simulink library "OpenManipulatorLib"  (R2017b)
settings: Solver=VariableStepAuto  StartTime=0.0  StopTime=10.0  RelTol=1e-3
undefined symbols (not defined in the file): ball_radius, eePositions, estDelay, filter_constant, gripper_force, initPosX, initPosY, initPosZ, initVelX, initVelY, initVelZ, polyOrder, time_jump, trajectoryPoints, Ts, wayPoints, X, Y, Z
libraries: sm_lib x85, nesl_utility x18, OpenManipulatorLib x11, fl_lib x4, Contact_Forces_Lib x3, dsppolyfun x2, Multibody_Multiphysics_Lib x2
(part 1 of 3)
settings Model: Creator=josea  LastModifiedBy=scastro

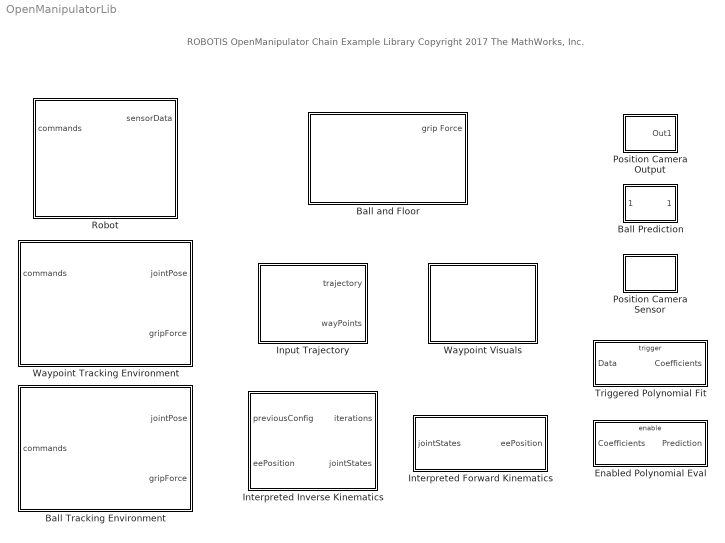
== system OpenManipulatorLib ==
  note: ROBOTIS OpenManipulator Chain Example Library
      |
      | Copyright 2017 The MathWorks, Inc.
  Ball Prediction : Subsystem  mask(Trajectory prediction in 2D){estDelay=estDelay, time_jump=time_jump, polyOrder=2}
      mask prompts: estDelay "Acquisition Window (seconds)"; time_jump "Time to look ahead (seconds)"; polyOrder "Polynomial Order"
      mask help: This subsystem estimates a polynomial using the data acquired until a specified time (estDelay), and then evaluates a polynomial with the calculated coefficients to give a rough prediction of where an object could be at a future point in time (time_jump).
      mask Display: image('PredictionIcon.png')
  Ball Tracking Environment : Subsystem  mask(Ball Tracking Environment){BallPositionY=-0.116, BallHeading=34.200, reverse=off, zVel=off}
      mask prompts: BallPositionY "Initial Ball Position (m)"; BallHeading "Initial Ball Heading (deg)"; reverse "Start from base and reverse heading"; zVel "3D Mode (Add Z initial velocity)"
      mask help: The initial position and velocity of the ball can be set to different conditions.
      mask init:
      | % Change the initial X position if the ball starting position is reversed
      | if ~reverse
      |     initPosX = 0.3;
      | else
      |     initPosX = 0;
      | end
      | 
      | % Initialize the ball velocity in XYZ coordinates
      | initPosY = BallPositionY;
      | VelocityMagnitude = 0.4;
      | initVelX = -1*VelocityMagnitude*cosd(BallHeading)*(-1)^reverse;
      | initVelY = VelocityMagnitude*sind(BallHeading);
      | initPosZ = 0.025;
      | if zVel
      |     initVelZ = 3.5;
      | else
      |     initVelZ = 0;
      | end
      mask Display: image('EnvironmentIcon.PNG')
  Ball and Floor : Subsystem  mask(Ball and Floor){PxPositionTargetValue=initPosX, PyPositionTargetValue=initPosY, PxVelocityTargetValue=initVelX, PyVelocityTargetValue=initVelY, PzPositionTargetValue=initPosZ, PzVelocityTargetValue=initVelZ}
      mask prompts: PxPositionTargetValue "Ball X Position Target"; PyPositionTargetValue "Ball Y Position Target"; PxVelocityTargetValue "Ball X Velocity Target"; PyVelocityTargetValue "Ball Y Velocity Target"; PzPositionTargetValue "Ball Z Position Target"; PzVelocityTargetValue "Ball Z Velocity Target"
      mask help: Subsystem containing ball and floor objects and the corresponding contact interfaces to interface with the manipulator gripper
      mask init:
      | if(any(PxVelocityTargetValue>0 || ...
      |        PyVelocityTargetValue>0 || ...
      |        PzVelocityTargetValue>0))
      |     stripColor = [1.0 0 1.0];
      | else
      |     stripColor = [0 0.6 0.6];
      | end
      mask TypeOptions PxPositionTargetValue: 6-DOF Joint/PxPositionTargetValue
      mask TypeOptions PyPositionTargetValue: 6-DOF Joint/PyPositionTargetValue
      mask TypeOptions PxVelocityTargetValue: 6-DOF Joint/PxVelocityTargetValue
      mask TypeOptions PyVelocityTargetValue: 6-DOF Joint/PyVelocityTargetValue
      mask TypeOptions PzPositionTargetValue: 6-DOF Joint/PzPositionTargetValue
      mask TypeOptions PzVelocityTargetValue: 6-DOF Joint/PzVelocityTargetValue
      mask Display: image('BallFloorIcon.png')
  Enabled Polynomial Eval : Subsystem
  Input Trajectory : Subsystem  mask(Input Trajectory){trajectorySelection=Simple}
      mask prompts: trajectorySelection "Trajectory type"
      mask help: This subsystem initializes data for the desired trajectory and waypoints. The necessary variables are created in the MATLAB workspace.
      mask init:
      | TS = get_param(gcb,'trajectorySelection');
      | switch TS
      |     case 'Simple'
      |         evalin('base','trajectorySelection=1;');
      |     case 'Complex'
      |         evalin('base','trajectorySelection=2;');
      |     case 'Gripper Fault'
      |         evalin('base','trajectorySelection=3;');
      | end
      | evalin('base','initOpenManipulatorWaypointTracking');
      mask TypeOptions trajectorySelection: Simple | Complex | Gripper Fault
      mask Display: image('wayPointsIcon.png')
  Interpreted Forward Kinematics : MATLAB Function  TreatAsAtomicUnit=on
  Interpreted Inverse Kinematics : MATLAB Function  TreatAsAtomicUnit=on
  Position Camera Output : Subsystem
      mask Display: image('CameraIcon.png')
  Position Camera Sensor : Subsystem
      mask Display: image('CameraIcon.png')
  Robot : Subsystem
      mask Display: image('RobotIcon.png')
  Triggered Polynomial Fit : Subsystem
  Waypoint Tracking Environment : Subsystem
      mask Display: image('EnvironmentWaypointsIcon.PNG')
  Waypoint Visuals : Subsystem  mask(Waypoint and Trajectory Visualization){spherePoints=wayPoints, sphereRadius=0.01, sphereColor=[0 0.5 1], splinePoints=trajectoryPoints, splineColor=[1 0 1]}
      mask prompts: spherePoints "Sphere Positions"; sphereRadius "Sphere Radius"; sphereColor "Sphere Color"; splinePoints "Trajectory Points"; splineColor "Trajectory Color"
      mask help:
      | This dynamic subsystem places spheres on the desired waypoints and visualizes a pre-computed trajectory as a 3D spline
      |
      | Sphere Positions and Trajectory Points are both vectors for which the first 3 columns correspond to the (X, Y, Z) coordinates of the waypoints or trajectory points.
      |
      | NOTE: Make sure the library link for the subsystem is broken when copied from the library. Otherwise the mask initialization will not be able to modify the subsystem contents.
      mask init:
      | % This initialization routine deletes everything within the mask except the
      | % inport and then rebuilds the subsystem with updated information from the
      | % mask parameters
      | 
      | subsystem = gcb;
      | blocks = find_system(subsystem,'LookUnderMasks','all');
      | 
      | % Delete all previous blocks except the inport
      | for idx = 2:length(blocks)-1
      |     delete_block(blocks{idx})
      | end
      | 
      | % Delete all signals
      | while ~isempty(find_system(subsystem,'LookUnderMasks','all','FindAll','on','type','line'))
      |     lines = find_system(subsystem,'LookUnderMasks','all','FindAll','on','type','line');
      |     delete_line(lines(1))
      | end
      | 
      | %%
      | pos1 = [140 100 180 140];
      | pos2 = [140 170 180 210];
      | 
      | set_param(strcat(subsystem,'/W'),'position',[140 60 180 80])
      | 
      | % Add spline to visualize trajectory
      | add_block('sm_lib/Curves and Surfaces/Spline',strcat(subsystem,'/Trajectory Spline'));
      | set_param(strcat(subsystem,'/Trajectory Spline'),'position',pos1,'Orientation','left');
      | set_param(strcat(subsystem,'/Trajectory Spline'),'DataPoints','splinePoints','EndCOnditionType','Natural','GraphicDiffuseColor','splineColor');
      | add_line(subsystem,strcat('W','/RConn1'),strcat('Trajectory Spline','/Lconn1'));
      | 
      | % Add waypoint sphere visuals
      | for idx = 1:size(spherePoints,1)
      |     pos1 = pos1 + [60 0 60 0];
      |     pos2 = pos2 + [60 0 60 0];
      |     
      |     % Add coordinate tranform and set parameters
      |     add_block('sm_lib/Frames and Transforms/Rigid Transform',strcat(subsystem,'/Rigid Transform',num2str(idx)));
      |     set_param(strcat(subsystem,'/Rigid Transform',num2str(idx)),'position',pos1,'Orientation','down');
      |     set_param(strcat(subsystem,'/Rigid Transform',num2str(idx)),'TranslationMethod','Cartesian','TranslationCartesianOffset',strcat('[',num2str(spherePoints(idx,1:3)),']'));
      |     add_line(subsystem,strcat('W','/RConn1'),strcat('Rigid Transform',num2str(idx),'/Lconn1'));
      |     
      |     % Add sphere ans set parameters
      |     add_block('sm_lib/Body Elements/Solid',strcat(subsystem,'/Solid',num2str(idx)))
      |     set_param(strcat(subsystem,'/Solid',num2str(idx)),'position',pos2,'GeometryShape','Sphere','GraphicDiffuseColor','sphereColor','SphereRadius','sphereRadius')
      |     add_line(subsystem,strcat('Rigid Transform',num2str(idx),'/Rconn1'),strcat('Solid',num2str(idx),'/RConn1'));
      |    
      | end
      mask DialogControl ParameterGroupVar Prompt: Sphere Parameters
      mask DialogControl Container3 Prompt: Spline Parameters
      mask Display: image('wayPointsIcon.png')

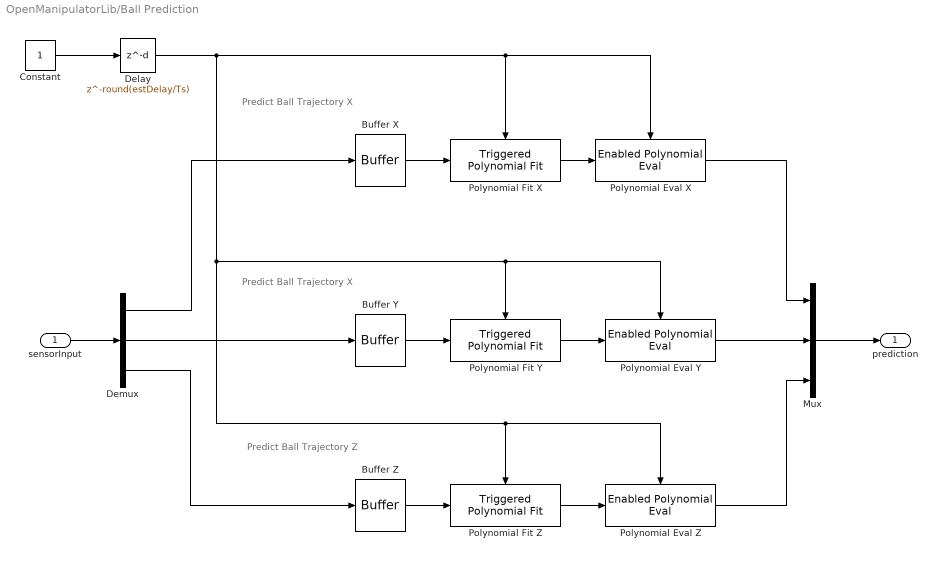
== system OpenManipulatorLib/Ball Prediction ==
  note: Predict Ball Trajectory X
  note: Predict Ball Trajectory X
  note: Predict Ball Trajectory Z
  sensorInput : Inport
  Buffer X : Buffer  N=round(estDelay/Ts)  V=round(estDelay/Ts)-1  OutputFrames=off
  Buffer Y : Buffer  N=round(estDelay/Ts)  V=round(estDelay/Ts)-1  OutputFrames=off
  Buffer Z : Buffer  N=round(estDelay/Ts)  V=round(estDelay/Ts)-1  OutputFrames=off
  Constant : Constant
  Delay : Delay  DelayLength=round(estDelay/Ts)
  Demux : Demux  Outputs=3
  Mux : Mux  Inputs=3
  Polynomial Eval X : OpenManipulatorLib/Enabled Polynomial Eval
  Polynomial Eval Y : OpenManipulatorLib/Enabled Polynomial Eval
  Polynomial Eval Z : OpenManipulatorLib/Enabled Polynomial Eval
  Polynomial Fit X : OpenManipulatorLib/Triggered Polynomial Fit
  Polynomial Fit Y : OpenManipulatorLib/Triggered Polynomial Fit
  Polynomial Fit Z : OpenManipulatorLib/Triggered Polynomial Fit
  prediction : Outport
  wires:
  Mux/1 -> prediction/1
  Constant/1 -> Delay/1
  sensorInput/1 -> Demux/1
  Demux/1 -> Buffer X/1
  Demux/2 -> Buffer Y/1
  Polynomial Eval X/1 -> Mux/1
  Delay/1 -> Polynomial Eval X/Enable, Polynomial Fit X/Trigger, Polynomial Eval Y/Enable, Polynomial Fit Y/Trigger, Polynomial Eval Z/Enable, Polynomial Fit Z/Trigger
  Polynomial Eval Z/1 -> Mux/3
  Demux/3 -> Buffer Z/1
  Buffer Z/1 -> Polynomial Fit Z/1
  Polynomial Fit Z/1 -> Polynomial Eval Z/1
  Polynomial Fit Y/1 -> Polynomial Eval Y/1
  Buffer Y/1 -> Polynomial Fit Y/1
  Buffer X/1 -> Polynomial Fit X/1
  Polynomial Fit X/1 -> Polynomial Eval X/1
  Polynomial Eval Y/1 -> Mux/2

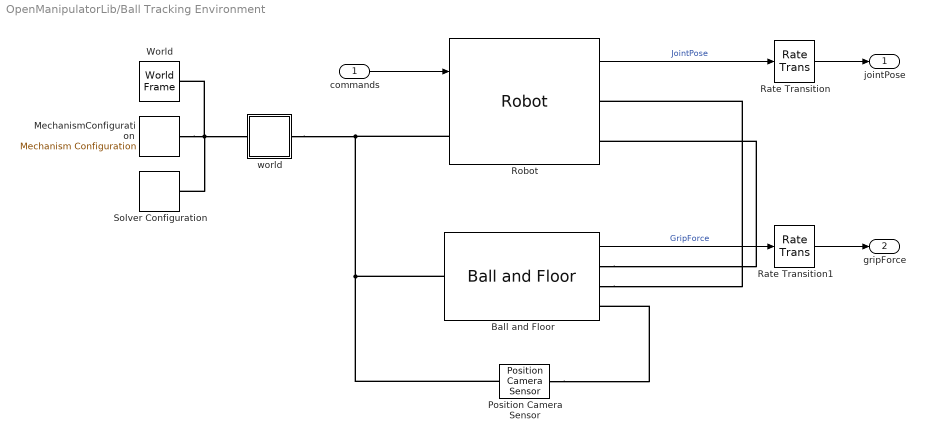
== system OpenManipulatorLib/Ball Tracking Environment ==
  commands : Inport
  Ball and Floor : OpenManipulatorLib/Ball and Floor  PxPositionTargetValue=initPosX  PyPositionTargetValue=initPosY  PxVelocityTargetValue=initVelX  PyVelocityTargetValue=initVelY  PzPositionTargetValue=initPosZ  PzVelocityTargetValue=initVelZ
  MechanismConfiguration : sm_lib/Utilities/Mechanism Configuration  UniformGravity=Constant  GravityVector=[0 0 -9.80665]  GravityUnits=m/s^2  LinearizationDelta=0.001
  Position Camera Sensor : OpenManipulatorLib/Position Camera Sensor  SystemSampleTime=-1
  Rate Transition : RateTransition
  Rate Transition1 : RateTransition
  Robot : OpenManipulatorLib/Robot  SystemSampleTime=-1
  Solver Configuration : nesl_utility/Solver Configuration  PhysicalDomain=network_engine_domain  SubClassName=solver  LeftPortType=input  RightPortType=generic  Accelerate=off  Tones=[]  Harmonics=[]  SimulateNoise=off  Profile=off  UseLocalSampling=off  EnableSwitchedLinearOptims=on  FrequencyDomain=off  UseCCode=off  RelTol=0.001  AbsTol=1e-06  MinStep=1e-09  ToWorkspace=off  RevertToSquareIcSolve=off  NumHomotopyIterations=100  PhasorMode=off  PhasorModeNumHarmonics=1  DoDC=off  ResidualTolerance=1e-09  UseLocalSolver=off  LocalSolverChoice=NE_BACKWARD_EULER_ADVANCER  LocalSolverSampleTime=0.001  DoFixedCost=off  MaxNonlinIter=3  MaxModeIter=2  LinearAlgebra=Sparse  DelaysMemoryBudget=1024  AutomaticFiltering=on  FilteringTimeConstant=0.001
  World : sm_lib/Frames and Transforms/World Frame
  world : Subsystem
  jointPose : Outport
  gripForce : Outport  Port=2
  wires:
  commands/1 -> Robot/1
  Robot/1 -> Rate Transition/1  "JointPose"
  Ball and Floor/1 -> Rate Transition1/1  "GripForce"
  Rate Transition/1 -> jointPose/1
  Rate Transition1/1 -> gripForce/1
  connections:
  World/RConn1 -- Solver Configuration/RConn1 -- world/LConn1 -- MechanismConfiguration/RConn1
  Position Camera Sensor/LConn1 -- Ball and Floor/LConn1 -- Robot/LConn1 -- world/RConn1
  Ball and Floor/RConn1 -- Robot/RConn2
  Ball and Floor/RConn2 -- Robot/RConn1
  Position Camera Sensor/RConn1 -- Ball and Floor/RConn3

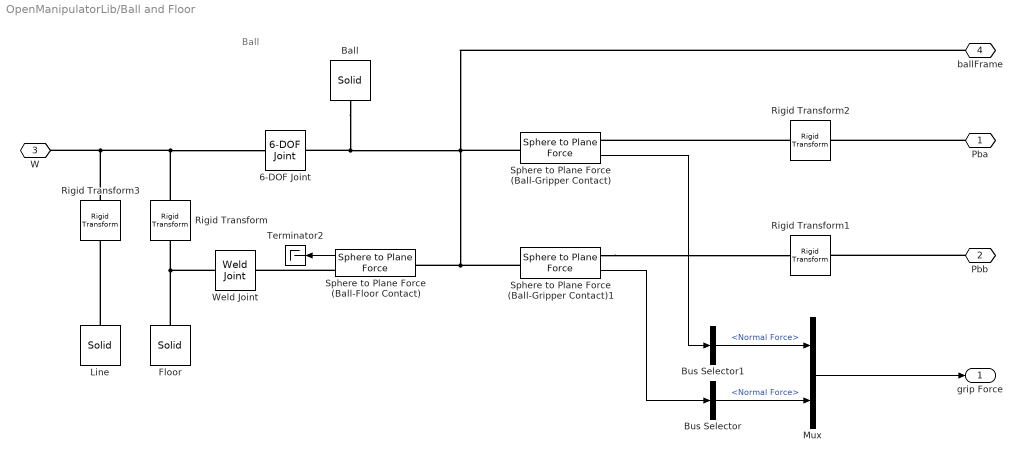
== system OpenManipulatorLib/Ball and Floor ==
  note: Ball
  6-DOF Joint : sm_lib/Joints/6-DOF Joint  SenseConstraintForce=off  SenseConstraintForceX=off  SenseConstraintForceY=off  SenseConstraintForceZ=off  SenseConstraintTorque=off  SenseConstraintTorqueX=off  SenseConstraintTorqueY=off  SenseConstraintTorqueZ=off  SenseTotalForce=off  SenseTotalForceX=off  SenseTotalForceY=off  SenseTotalForceZ=off  SenseTotalTorque=off  SenseTotalTorqueX=off  SenseTotalTorqueY=off  SenseTotalTorqueZ=off  CompositeWrenchDir=FollowerOnBase  CompositeWrenchFrame=BaseFrame  PxEquilibriumPosition=0  PxEquilibriumPositionUnits=m  PxSpringStiffness=0  PxSpringStiffnessUnits=N/m  PxDampingCoefficient=contact_floor.dampingCoeff  PxDampingCoefficientUnits=N/(m/s)  PxTorqueActuationMode=NoTorque  PxMotionActuationMode=ComputedMotion  PxSensePosition=off  PxSenseVelocity=off  PxSenseAcceleration=off  PxSenseTorqueForce=off  PxPositionTargetSpecify=on  PxPositionTargetPriority=High  PxPositionTargetValue=PxPositionTargetValue  PxPositionTargetValueUnits=m  PxVelocityTargetSpecify=on  PxVelocityTargetPriority=High  PxVelocityTargetValue=PxVelocityTargetValue  PxVelocityTargetValueUnits=m/s  PyEquilibriumPosition=0  PyEquilibriumPositionUnits=m  PySpringStiffness=0  PySpringStiffnessUnits=N/m  PyDampingCoefficient=contact_floor.dampingCoeff  PyDampingCoefficientUnits=N/(m/s)  PyTorqueActuationMode=NoTorque  PyMotionActuationMode=ComputedMotion  PySensePosition=off  PySenseVelocity=off  PySenseAcceleration=off  PySenseTorqueForce=off  PyPositionTargetSpecify=on  PyPositionTargetPriority=High  PyPositionTargetValue=PyPositionTargetValue  PyPositionTargetValueUnits=m  PyVelocityTargetSpecify=on  PyVelocityTargetPriority=High  PyVelocityTargetValue=PyVelocityTargetValue  PyVelocityTargetValueUnits=m/s  PzEquilibriumPosition=0  PzEquilibriumPositionUnits=m  PzSpringStiffness=0  PzSpringStiffnessUnits=N/m  PzDampingCoefficient=0  PzDampingCoefficientUnits=N/(m/s)  PzTorqueActuationMode=NoTorque  PzMotionActuationMode=ComputedMotion  PzSensePosition=off  PzSenseVelocity=off  PzSenseAcceleration=off  PzSenseTorqueForce=off  PzPositionTargetSpecify=on  PzPositionTargetPriority=High  PzPositionTargetValue=PzPositionTargetValue  PzPositionTargetValueUnits=m  PzVelocityTargetSpecify=on  PzVelocityTargetPriority=High  PzVelocityTargetValue=PzVelocityTargetValue  PzVelocityTargetValueUnits=m/s  SphDefPosRotationMethod=None  SphDefPosRotationAngleUnits=deg  SphDefPosRotationStandardAxis=+Z  SphDefPosRotationAngle=0.0  SphDefPosRotationArbitraryAxis=[0 0 1]  SphDefPosFollAlignAxisA=+X  SphDefPosBaseAlignAxisA=+Y  SphDefPosFollAlignAxisB=+Y  SphDefPosBaseAlignAxisB=+Z  SphDefPosRotationSequenceAxes=FollowerAxes  SphDefPosRotationSequence=XYX  SphDefPosRotationSequenceAngles=[0 0 0]  SphDefPosRotationSequenceAnglesUnits=deg  SphDefPosRotationMatrix=[1 0 0; 0 1 0; 0 0 1]  SphEqPosRotationMethod=None  SphEqPosRotationAngleUnits=deg  SphEqPosRotationStandardAxis=+Z  SphEqPosRotationAngle=0.0  SphEqPosRotationArbitraryAxis=[0 0 1]  SphEqPosFollAlignAxisA=+X  SphEqPosBaseAlignAxisA=+Y  SphEqPosFollAlignAxisB=+Y  SphEqPosBaseAlignAxisB=+Z  SphEqPosRotationSequenceAxes=FollowerAxes  SphEqPosRotationSequence=XYX  SphEqPosRotationSequenceAngles=[0 0 0]  SphEqPosRotationSequenceAnglesUnits=deg  SphEqPosRotationMatrix=[1 0 0; 0 1 0; 0 0 1]  SphSpringStiffness=0  SphSpringStiffnessUnits=N*m/deg  SphDampingCoefficient=contact_floor.dampingCoeffR  SphDampingCoefficientUnits=N*m/(rad/s)  SphActuateTorqueX=off  SphActuateTorqueY=off  SphActuateTorqueZ=off  SphActuateTorque=off  SphTorqueActuationMode=NoTorque  SphMotionActuationMode=ComputedMotion  SphActuationFrame=BaseFrame  SphSensePosition=off  SphSenseVelocityX=off  SphSenseVelocityY=off  SphSenseVelocityZ=off  SphSenseVelocity=off  SphSenseAccelerationX=off  SphSenseAccelerationY=off  SphSenseAccelerationZ=off  SphSenseAcceleration=off  SphSenseTorqueX=off  SphSenseTorqueY=off  SphSenseTorqueZ=off  SphSenseTorqueForce=off  SphSensingFrame=BaseFrame  SphPositionTargetRotationMethod=None  SphPositionTargetRotationAngleUnits=deg  SphPositionTargetRotationStandardAxis=+Z  SphPositionTargetRotationAngle=0.0  SphPositionTargetRotationArbitraryAxis=[0 0 1]  SphPositionTargetFollAlignAxisA=+X  SphPositionTargetBaseAlignAxisA=+Y  SphPositionTargetFollAlignAxisB=+Y  SphPositionTargetBaseAlignAxisB=+Z  SphPositionTargetRotationSequenceAxes=FollowerAxes  SphPositionTargetRotationSequence=XYX  SphPositionTargetRotationSequenceAngles=[0 0 0]  SphPositionTargetRotationSequenceAnglesUnits=deg  SphPositionTargetRotationMatrix=[1 0 0; 0 1 0; 0 0 1]  SphPositionTargetSpecify=off  SphPositionTargetPriority=High  SphVelocityTargetValue=[0 0 0]  SphVelocityTargetValueUnits=deg/s  SphVelocityTargetSpecify=off  SphVelocityTargetPriority=High  SphVelocityTargetInFollowerFrame=on
  Ball : sm_lib/Body Elements/Solid  InertiaType=CalculateFromGeometry  Mass=0.01  MassUnits=kg  CenterOfMass=[0 0 0]  CenterOfMassUnits=m  MomentsOfInertia=[1 1 1]  MomentsOfInertiaUnits=kg*m^2  ProductsOfInertia=[1 1 1]  ProductsOfInertiaUnits=kg*m^2  DensityBased=off  Density=1000  DensityUnits=kg/m^3  DoExposeReferenceFrame=on  SerializedFrames=<Frames/>  GraphicType=FromGeometry  MarkerShape=Sphere  MarkerSize=10  GraphicVisPropType=SimpleVisualProperties  GraphicDiffuseColor=[1.0 0.2 0.2]  GraphicSpecularColor=[0.5 0.5 0.5 1.0]  GraphicAmbientColor=[0.15 0.15 0.15 1.0]  GraphicEmissiveColor=[0.0 0.0 0.0 1.0]  GraphicShininess=75  GraphicOpacity=1.0  GeometryShape=Sphere  RectangleSize=[1 1]  RectangleSizeUnits=m  BrickDimensions=[40 40 0.5]  BrickDimensionUnits=cm  CylinderRadius=1  CylinderRadiusUnits=m  CylinderLength=1  CylinderLengthUnits=m  SphereRadius=ball_radius  SphereRadiusUnits=cm  EllipsoidRadii=[1 1 1]  EllipsoidRadiiUnits=m  ExtrusionCrossSection=[1 1; -1 1; -1 -1; 1 -1]  ExtrusionCrossSectionUnits=m  ExtrusionLength=1  ExtrusionLengthUnits=m  PolygonNumSides=3  PolygonOuterRadius=1  PolygonOuterRadiusUnits=m  ExtGeomFileType=STEP  ExtGeomFileUnits=m  RevolutionCrossSection=[1 1; 1 -1; 2 -1; 2 1]  RevolutionCrossSectionUnits=m  RevolutionExtent=Full  RevolutionAngle=180  RevolutionAngleUnits=deg
  Bus Selector : BusSelector  OutputSignals=Normal Force
  Bus Selector1 : BusSelector  OutputSignals=Normal Force
  Floor : sm_lib/Body Elements/Solid  InertiaType=CalculateFromGeometry  Mass=1  MassUnits=kg  CenterOfMass=[0 0 0]  CenterOfMassUnits=m  MomentsOfInertia=[1 1 1]  MomentsOfInertiaUnits=kg*m^2  ProductsOfInertia=[1 1 1]  ProductsOfInertiaUnits=kg*m^2  DensityBased=on  Density=1000  DensityUnits=kg/m^3  DoExposeReferenceFrame=on  SerializedFrames=<Frames/>  GraphicType=FromGeometry  MarkerShape=Sphere  MarkerSize=10  GraphicVisPropType=SimpleVisualProperties  GraphicDiffuseColor=[0.0 0.6 0.6]  GraphicSpecularColor=[0.5 0.5 0.5 1.0]  GraphicAmbientColor=[0.15 0.15 0.15 1.0]  GraphicEmissiveColor=[0.0 0.0 0.0 1.0]  GraphicShininess=75  GraphicOpacity=1.0  GeometryShape=Brick  RectangleSize=[1 1]  RectangleSizeUnits=m  BrickDimensions=floor_dimensions  BrickDimensionUnits=cm  CylinderRadius=1  CylinderRadiusUnits=m  CylinderLength=1  CylinderLengthUnits=m  SphereRadius=1  SphereRadiusUnits=m  EllipsoidRadii=[1 1 1]  EllipsoidRadiiUnits=m  ExtrusionCrossSection=[1 1; -1 1; -1 -1; 1 -1]  ExtrusionCrossSectionUnits=m  ExtrusionLength=1  ExtrusionLengthUnits=m  PolygonNumSides=3  PolygonOuterRadius=1  PolygonOuterRadiusUnits=m  ExtGeomFileType=STEP  ExtGeomFileUnits=m  RevolutionCrossSection=[1 1; 1 -1; 2 -1; 2 1]  RevolutionCrossSectionUnits=m  RevolutionExtent=Full  RevolutionAngle=180  RevolutionAngleUnits=deg
  Line : sm_lib/Body Elements/Solid  InertiaType=CalculateFromGeometry  Mass=1  MassUnits=kg  CenterOfMass=[0 0 0]  CenterOfMassUnits=m  MomentsOfInertia=[1 1 1]  MomentsOfInertiaUnits=kg*m^2  ProductsOfInertia=[1 1 1]  ProductsOfInertiaUnits=kg*m^2  DensityBased=on  Density=1000  DensityUnits=kg/m^3  DoExposeReferenceFrame=on  SerializedFrames=<Frames/>  GraphicType=FromGeometry  MarkerShape=Sphere  MarkerSize=10  GraphicVisPropType=SimpleVisualProperties  GraphicDiffuseColor=stripColor  GraphicSpecularColor=[0.5 0.5 0.5 1.0]  GraphicAmbientColor=[0.15 0.15 0.15 1.0]  GraphicEmissiveColor=[0.0 0.0 0.0 1.0]  GraphicShininess=75  GraphicOpacity=1.0  GeometryShape=Brick  RectangleSize=[1 1]  RectangleSizeUnits=m  BrickDimensions=[1 40 0.505]  BrickDimensionUnits=cm  CylinderRadius=1  CylinderRadiusUnits=m  CylinderLength=1  CylinderLengthUnits=m  SphereRadius=1  SphereRadiusUnits=m  EllipsoidRadii=[1 1 1]  EllipsoidRadiiUnits=m  ExtrusionCrossSection=[1 1; -1 1; -1 -1; 1 -1]  ExtrusionCrossSectionUnits=m  ExtrusionLength=1  ExtrusionLengthUnits=m  PolygonNumSides=3  PolygonOuterRadius=1  PolygonOuterRadiusUnits=m  ExtGeomFileType=STEP  ExtGeomFileUnits=m  RevolutionCrossSection=[1 1; 1 -1; 2 -1; 2 1]  RevolutionCrossSectionUnits=m  RevolutionExtent=Full  RevolutionAngle=180  RevolutionAngleUnits=deg
  Mux : Mux  Inputs=2
  Rigid Transform : sm_lib/Frames and Transforms/Rigid Transform  TranslationMethod=Cartesian  TranslationStandardOffset=0  TranslationLengthUnit=cm  TranslationStandardAxis=+Z  TranslationCartesianOffset=[15 0 -0.25]  TranslationROffset=0  TranslationROffsetUnits=m  TranslationZOffset=0  TranslationZOffsetUnits=m  TranslationThetaOffset=0  TranslationThetaOffsetUnits=deg  RotationMethod=None  RotationAngleUnits=deg  RotationStandardAxis=+Z  RotationAngle=0.0  RotationArbitraryAxis=[0 0 1]  FollAlignAxisA=+X  BaseAlignAxisA=+Y  FollAlignAxisB=+Y  BaseAlignAxisB=+Z  RotationSequenceAxes=FollowerAxes  RotationSequence=XYX  RotationSequenceAngles=[0 0 0]  RotationSequenceAnglesUnits=deg  RotationMatrix=[1 0 0; 0 1 0; 0 0 1]
  Rigid Transform1 : sm_lib/Frames and Transforms/Rigid Transform  TranslationMethod=None  TranslationStandardOffset=0  TranslationLengthUnit=cm  TranslationStandardAxis=+Z  TranslationCartesianOffset=[15 0 -0.25]  TranslationROffset=0  TranslationROffsetUnits=m  TranslationZOffset=0  TranslationZOffsetUnits=m  TranslationThetaOffset=0  TranslationThetaOffsetUnits=deg  RotationMethod=StandardAxis  RotationAngleUnits=deg  RotationStandardAxis=+X  RotationAngle=-90  RotationArbitraryAxis=[0 0 1]  FollAlignAxisA=+X  BaseAlignAxisA=+Y  FollAlignAxisB=+Y  BaseAlignAxisB=+Z  RotationSequenceAxes=FollowerAxes  RotationSequence=XYX  RotationSequenceAngles=[0 0 0]  RotationSequenceAnglesUnits=deg  RotationMatrix=[1 0 0; 0 1 0; 0 0 1]
  Rigid Transform2 : sm_lib/Frames and Transforms/Rigid Transform  TranslationMethod=None  TranslationStandardOffset=0  TranslationLengthUnit=cm  TranslationStandardAxis=+Z  TranslationCartesianOffset=[15 0 -0.25]  TranslationROffset=0  TranslationROffsetUnits=m  TranslationZOffset=0  TranslationZOffsetUnits=m  TranslationThetaOffset=0  TranslationThetaOffsetUnits=deg  RotationMethod=StandardAxis  RotationAngleUnits=deg  RotationStandardAxis=+X  RotationAngle=-90  RotationArbitraryAxis=[0 0 1]  FollAlignAxisA=+X  BaseAlignAxisA=+Y  FollAlignAxisB=+Y  BaseAlignAxisB=+Z  RotationSequenceAxes=FollowerAxes  RotationSequence=XYX  RotationSequenceAngles=[0 0 0]  RotationSequenceAnglesUnits=deg  RotationMatrix=[1 0 0; 0 1 0; 0 0 1]
  Rigid Transform3 : sm_lib/Frames and Transforms/Rigid Transform  TranslationMethod=Cartesian  TranslationStandardOffset=0  TranslationLengthUnit=cm  TranslationStandardAxis=+Z  TranslationCartesianOffset=[30 0 -0.25]  TranslationROffset=0  TranslationROffsetUnits=m  TranslationZOffset=0  TranslationZOffsetUnits=m  TranslationThetaOffset=0  TranslationThetaOffsetUnits=deg  RotationMethod=None  RotationAngleUnits=deg  RotationStandardAxis=+Z  RotationAngle=0.0  RotationArbitraryAxis=[0 0 1]  FollAlignAxisA=+X  BaseAlignAxisA=+Y  FollAlignAxisB=+Y  BaseAlignAxisB=+Z  RotationSequenceAxes=FollowerAxes  RotationSequence=XYX  RotationSequenceAngles=[0 0 0]  RotationSequenceAnglesUnits=deg  RotationMatrix=[1 0 0; 0 1 0; 0 0 1]
  Sphere to Plane Force (Ball-Floor Contact) : Contact_Forces_Lib/3D/Sphere to Plane Force  sphere_rad=ball_radius*0.01  plane_lenx=contact_floor.planeLength  plane_leny=contact_floor.planeLength  plane_depth=contact_floor.planeDepth  force_law=Linear  k_contact=contact_floor.stiffness  b_contact=contact_floor.damping  pen_full_damp_F=1e-4  pen_exponent=2  custom_param_1=1  custom_param_2=1  friction_law=Stick-Slip Continuous  mu_kinetic=contact_floor.kFrictionCoeff  mu_static=contact_floor.sFrictionCoeff  v_thr=0.01  vis_on=off  vis_opc_en=0  vis_len_plaBz=0.005  vis_clr=[0.9 0.2 0.2]  vis_opc=0.7
  Sphere to Plane Force (Ball-Gripper Contact) : Contact_Forces_Lib/3D/Sphere to Plane Force  sphere_rad=ball_radius*0.01  plane_lenx=contact_gripper.planeLength_x  plane_leny=contact_gripper.planeLength_y  plane_depth=contact_gripper.planeDepth  force_law=Linear  k_contact=contact_gripper.stiffness  b_contact=contact_gripper.damping  pen_full_damp_F=1e-4  pen_exponent=1  custom_param_1=1  custom_param_2=1  friction_law=Stick-Slip Continuous  mu_kinetic=contact_gripper.kFrictionCoeff  mu_static=contact_gripper.sFrictionCoeff  v_thr=0.01  vis_on=off  vis_opc_en=0  vis_len_plaBz=0.005  vis_clr=[0.9 0.2 0.2]  vis_opc=0.7
  Sphere to Plane Force (Ball-Gripper Contact)1 : Contact_Forces_Lib/3D/Sphere to Plane Force  sphere_rad=ball_radius*0.01  plane_lenx=contact_gripper.planeLength_x  plane_leny=contact_gripper.planeLength_y  plane_depth=contact_gripper.planeDepth  force_law=Linear  k_contact=contact_gripper.stiffness  b_contact=contact_gripper.damping  pen_full_damp_F=1e-4  pen_exponent=1  custom_param_1=1  custom_param_2=1  friction_law=Stick-Slip Continuous  mu_kinetic=contact_gripper.kFrictionCoeff  mu_static=contact_gripper.sFrictionCoeff  v_thr=0.01  vis_on=off  vis_opc_en=0  vis_len_plaBz=0.005  vis_clr=[0.9 0.2 0.2]  vis_opc=0.7
  Terminator2 : Terminator
  Weld Joint : sm_lib/Joints/Weld Joint  SenseConstraintForce=off  SenseConstraintForceX=off  SenseConstraintForceY=off  SenseConstraintForceZ=off  SenseConstraintTorque=off  SenseConstraintTorqueX=off  SenseConstraintTorqueY=off  SenseConstraintTorqueZ=off  SenseTotalForce=off  SenseTotalForceX=off  SenseTotalForceY=off  SenseTotalForceZ=off  SenseTotalTorque=off  SenseTotalTorqueX=off  SenseTotalTorqueY=off  SenseTotalTorqueZ=off  CompositeWrenchDir=FollowerOnBase  CompositeWrenchFrame=BaseFrame
  Pba : PMIOPort  Port=1  Side=Right
  Pbb : PMIOPort  Port=2  Side=Right
  W : PMIOPort  Port=3  Side=Left
  ballFrame : PMIOPort  Port=4  Side=Right
  grip Force : Outport
  wires:
  Sphere to Plane Force (Ball-Gripper Contact)1/1 -> Bus Selector/1
  Sphere to Plane Force (Ball-Floor Contact)/1 -> Terminator2/1
  Sphere to Plane Force (Ball-Gripper Contact)/1 -> Bus Selector1/1
  Bus Selector1/1 -> Mux/1  "<Normal Force>"
  Bus Selector/1 -> Mux/2  "<Normal Force>"
  Mux/1 -> grip Force/1
  connections:
  Floor/RConn1 -- Weld Joint/LConn1 -- Rigid Transform/RConn1
  Pba/RConn1 -- Rigid Transform2/LConn1
  6-DOF Joint/RConn1 -- Sphere to Plane Force (Ball-Gripper Contact)/LConn1 -- ballFrame/RConn1 -- Sphere to Plane Force (Ball-Gripper Contact)1/LConn1 -- Sphere to Plane Force (Ball-Floor Contact)/LConn1 -- Ball/RConn1
  Pbb/RConn1 -- Rigid Transform1/LConn1
  Sphere to Plane Force (Ball-Gripper Contact)1/RConn1 -- Rigid Transform1/RConn1
  Sphere to Plane Force (Ball-Floor Contact)/RConn1 -- Weld Joint/RConn1
  Rigid Transform2/RConn1 -- Sphere to Plane Force (Ball-Gripper Contact)/RConn1
  Rigid Transform/LConn1 -- Rigid Transform3/LConn1 -- W/RConn1 -- 6-DOF Joint/LConn1
  Line/RConn1 -- Rigid Transform3/RConn1

== system OpenManipulatorLib/Enabled Polynomial Eval ==
  Coefficients : Inport
  Enable : EnablePort
  Add : Sum
  Clock : Clock
  Constant : Constant  Value=time_jump
  Polynomial Evaluation : dsppolyfun/Polynomial Evaluation  useConstCoeffs=off  constCoeffs=[5 4 3 2 1]
      settings: SourceProductName=DSP System Toolbox  SourceProductBaseCode=DS
  Rate Transition : RateTransition  OutPortSampleTime=Ts
  Prediction : Outport
  wires:
  Polynomial Evaluation/1 -> Prediction/1
  Add/1 -> Polynomial Evaluation/1
  Constant/1 -> Add/2
  Rate Transition/1 -> Add/1
  Coefficients/1 -> Polynomial Evaluation/2
  Clock/1 -> Rate Transition/1

== system OpenManipulatorLib/Input Trajectory ==
  Constant : Constant  Value=eePositions
  Constant3 : Constant  Value=wayPoints
  trajectory : Outport
  wayPoints : Outport  Port=2
  wires:
  Constant/1 -> trajectory/1
  Constant3/1 -> wayPoints/1

== system OpenManipulatorLib/Position Camera Output ==
  Mux : Mux  Inputs=3
  Out1 : Outport
  wires:
  [ballX] -> Mux/1
  [ballY] -> Mux/2
  Mux/1 -> Out1/1
  [ballZ] -> Mux/3

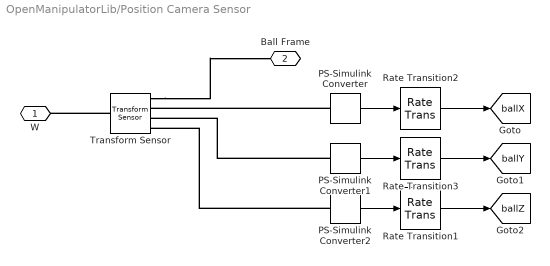
== system OpenManipulatorLib/Position Camera Sensor ==
  PS-Simulink Converter : nesl_utility/PS-Simulink Converter  PhysicalDomain=network_engine_domain  SubClassName=ps_output  LeftPortType=input  RightPortType=output  PseudoPeriodic=off  Frequencies=[]  Unit=1  AffineConversion=off
  PS-Simulink Converter1 : nesl_utility/PS-Simulink Converter  PhysicalDomain=network_engine_domain  SubClassName=ps_output  LeftPortType=input  RightPortType=output  PseudoPeriodic=off  Frequencies=[]  Unit=1  AffineConversion=off
  PS-Simulink Converter2 : nesl_utility/PS-Simulink Converter  PhysicalDomain=network_engine_domain  SubClassName=ps_output  LeftPortType=input  RightPortType=output  PseudoPeriodic=off  Frequencies=[]  Unit=1  AffineConversion=off
  Rate Transition1 : RateTransition  OutPortSampleTime=Ts
  Rate Transition2 : RateTransition  OutPortSampleTime=Ts
  Rate Transition3 : RateTransition  OutPortSampleTime=Ts
  Transform Sensor : sm_lib/Frames and Transforms/Transform Sensor  MeasurementFrame=World  SenseAngle=off  SenseAxis=off  SenseAngle1=off  SenseAngle2=off  SenseAngle3=off  SenseQ=off  SenseR=off  SenseOmegaX=off  SenseOmegaY=off  SenseOmegaZ=off  SenseOmega1=off  SenseOmega2=off  SenseOmega3=off  SenseQDot=off  SenseRDot=off  SenseAlphaX=off  SenseAlphaY=off  SenseAlphaZ=off  SenseAlpha1=off  SenseAlpha2=off  SenseAlpha3=off  SenseQDDot=off  SenseRDDot=off  SenseX=on  SenseY=on  SenseZ=on  SenseRad=off  SenseAzim=off  SenseDist=off  SenseInc=off  SenseXDot=off  SenseYDot=off  SenseZDot=off  SenseRadDot=off  SenseAzimDot=off  SenseDistDot=off  SenseIncDot=off  SenseXDDot=off  SenseYDDot=off  SenseZDDot=off  SenseRadDDot=off  SenseAzimDDot=off  SenseDistDDot=off  SenseIncDDot=off
  W : PMIOPort  Port=1  Side=Left
  Ball Frame : PMIOPort  Port=2  Side=Right
  tag scope: ballX=global, ballY=global, ballZ=global
  wires:
  PS-Simulink Converter1/1 -> Rate Transition3/1
  PS-Simulink Converter/1 -> Rate Transition2/1
  Rate Transition2/1 -> [ballX]
  Rate Transition3/1 -> [ballY]
  Rate Transition1/1 -> [ballZ]
  PS-Simulink Converter2/1 -> Rate Transition1/1
  connections:
  PS-Simulink Converter/LConn1 -- Transform Sensor/RConn2
  PS-Simulink Converter1/LConn1 -- Transform Sensor/RConn3
  Transform Sensor/LConn1 -- W/RConn1
  Transform Sensor/RConn1 -- Ball Frame/RConn1
  PS-Simulink Converter2/LConn1 -- Transform Sensor/RConn4

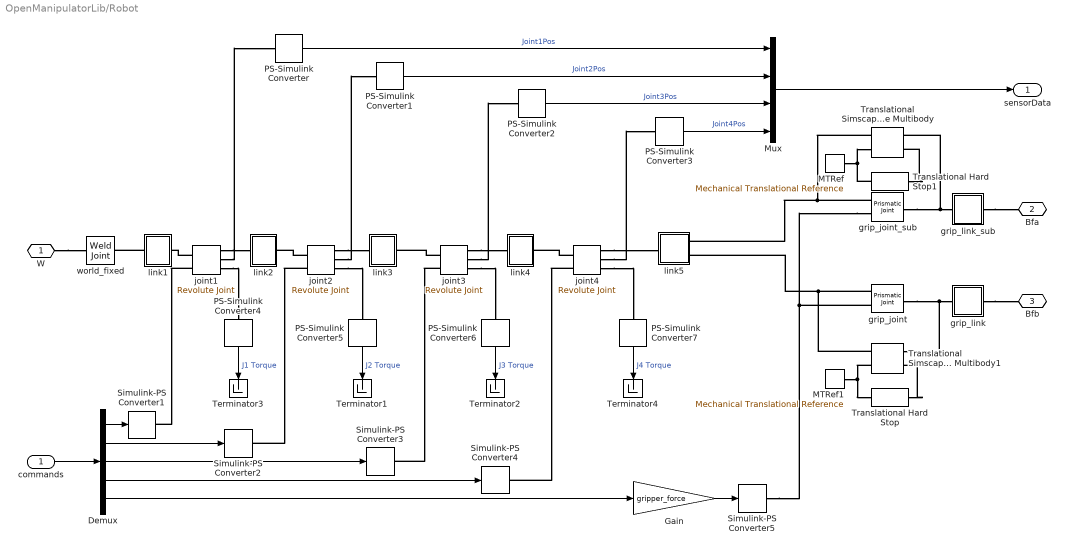
== system OpenManipulatorLib/Robot ==
  commands : Inport
  Demux : Demux  Outputs=5
  Gain : Gain  Gain=gripper_force
  MTRef : fl_lib/Mechanical/Translational Elements/Mechanical Translational Reference
  MTRef1 : fl_lib/Mechanical/Translational Elements/Mechanical Translational Reference
  Mux : Mux
  PS-Simulink Converter{,1..7} (8 alike) : nesl_utility/PS-Simulink Converter  PhysicalDomain=network_engine_domain  SubClassName=ps_output  LeftPortType=input  RightPortType=output  PseudoPeriodic=off  Frequencies=[]  Unit=1  AffineConversion=off
  Simulink-PS Converter{1..4} (4 alike) : nesl_utility/Simulink-PS Converter  PhysicalDomain=network_engine_domain  SubClassName=ps_input  LeftPortType=input  RightPortType=output  PseudoPeriodic=off  Frequencies=[]  NoiseDistribution=none  NoiseParameters=[]  Unit=1  AffineConversion=off  FilteringAndDerivatives=filter  SimscapeFilterOrder=2  InputFilterTimeConstant=filter_constant  UdotUserProvided=0
  Simulink-PS Converter5 : nesl_utility/Simulink-PS Converter  PhysicalDomain=network_engine_domain  SubClassName=ps_input  LeftPortType=input  RightPortType=output  PseudoPeriodic=off  Frequencies=[]  NoiseDistribution=none  NoiseParameters=[]  Unit=1  AffineConversion=off  FilteringAndDerivatives=filter  SimscapeFilterOrder=2  InputFilterTimeConstant=filter_constant*0.1  UdotUserProvided=0
  Terminator{1..4} (4 alike) : Terminator
  Translational Simscape Multibody : Multibody_Multiphysics_Lib/Interfaces/Translational Simscape Multibody
      settings: SourceProductName=Simscape Multibody Multiphysics Library
  Translational Simscape Multibody1 : Multibody_Multiphysics_Lib/Interfaces/Translational Simscape Multibody
      settings: SourceProductName=Simscape Multibody Multiphysics Library
  Translational Hard Stop : fl_lib/Mechanical/Translational Elements/Translational Hard Stop  upper_bnd=0.01 m  lower_bnd=-0.03 m  stiff_up=1e6 N/m  stiff_low=1e6 N/m  D_up=150 N/(m/s)  D_low=150 N/(m/s)  model=1  transition=0.1 mm  v_specify=off  v_priority=None  v=0 m/s  v_nominal_specify=off  v_nominal_unit=m/s  v_nominal_value=1  f_specify=off  f_priority=None  f=0 N  f_nominal_specify=off  f_nominal_unit=N  f_nominal_value=1  x_specify=off  x_priority=High  x=0 m  x_nominal_specify=off  x_nominal_unit=m  x_nominal_value=1
  Translational Hard Stop1 : fl_lib/Mechanical/Translational Elements/Translational Hard Stop  upper_bnd=0.01 m  lower_bnd=-0.03 m  stiff_up=1e6 N/m  stiff_low=1e6 N/m  D_up=150 N/(m/s)  D_low=150 N/(m/s)  model=1  transition=0.1 mm  v_specify=off  v_priority=None  v=0 m/s  v_nominal_specify=off  v_nominal_unit=m/s  v_nominal_value=1  f_specify=off  f_priority=None  f=0 N  f_nominal_specify=off  f_nominal_unit=N  f_nominal_value=1  x_specify=off  x_priority=High  x=0 m  x_nominal_specify=off  x_nominal_unit=m  x_nominal_value=1
  grip_joint : sm_lib/Joints/Prismatic Joint  SenseConstraintForce=off  SenseConstraintForceX=off  SenseConstraintForceY=off  SenseConstraintForceZ=off  SenseConstraintTorque=off  SenseConstraintTorqueX=off  SenseConstraintTorqueY=off  SenseConstraintTorqueZ=off  SenseTotalForce=off  SenseTotalForceX=off  SenseTotalForceY=off  SenseTotalForceZ=off  SenseTotalTorque=off  SenseTotalTorqueX=off  SenseTotalTorqueY=off  SenseTotalTorqueZ=off  CompositeWrenchDir=FollowerOnBase  CompositeWrenchFrame=BaseFrame  EquilibriumPosition=0  EquilibriumPositionUnits=m  SpringStiffness=1  SpringStiffnessUnits=N/m  DampingCoefficient=5  DampingCoefficientUnits=kg/s  TorqueActuationMode=InputTorque  MotionActuationMode=ComputedMotion  SensePosition=off  SenseVelocity=off  SenseAcceleration=off  SenseTorqueForce=off  PositionTargetSpecify=off  PositionTargetPriority=High  PositionTargetValue=0  PositionTargetValueUnits=m  VelocityTargetSpecify=off  VelocityTargetPriority=High  VelocityTargetValue=0  VelocityTargetValueUnits=m/s
  grip_joint_sub : sm_lib/Joints/Prismatic Joint  SenseConstraintForce=off  SenseConstraintForceX=off  SenseConstraintForceY=off  SenseConstraintForceZ=off  SenseConstraintTorque=off  SenseConstraintTorqueX=off  SenseConstraintTorqueY=off  SenseConstraintTorqueZ=off  SenseTotalForce=off  SenseTotalForceX=off  SenseTotalForceY=off  SenseTotalForceZ=off  SenseTotalTorque=off  SenseTotalTorqueX=off  SenseTotalTorqueY=off  SenseTotalTorqueZ=off  CompositeWrenchDir=FollowerOnBase  CompositeWrenchFrame=BaseFrame  EquilibriumPosition=0  EquilibriumPositionUnits=m  SpringStiffness=1  SpringStiffnessUnits=N/m  DampingCoefficient=5  DampingCoefficientUnits=kg/s  TorqueActuationMode=InputTorque  MotionActuationMode=ComputedMotion  SensePosition=off  SenseVelocity=off  SenseAcceleration=off  SenseTorqueForce=off  PositionTargetSpecify=off  PositionTargetPriority=High  PositionTargetValue=0  PositionTargetValueUnits=m  VelocityTargetSpecify=off  VelocityTargetPriority=High  VelocityTargetValue=0  VelocityTargetValueUnits=m/s
  grip_link : Subsystem
  grip_link_sub : Subsystem
  joint{1..4} (4 alike) : sm_lib/Joints/Revolute Joint  SenseConstraintForce=off  SenseConstraintForceX=off  SenseConstraintForceY=off  SenseConstraintForceZ=off  SenseConstraintTorque=off  SenseConstraintTorqueX=off  SenseConstraintTorqueY=off  SenseConstraintTorqueZ=off  SenseTotalForce=off  SenseTotalForceX=off  SenseTotalForceY=off  SenseTotalForceZ=off  SenseTotalTorque=off  SenseTotalTorqueX=off  SenseTotalTorqueY=off  SenseTotalTorqueZ=off  CompositeWrenchDir=FollowerOnBase  CompositeWrenchFrame=BaseFrame  EquilibriumPosition=0  EquilibriumPositionUnits=deg  SpringStiffness=0  SpringStiffnessUnits=N*m/deg  DampingCoefficient=joint_damping  DampingCoefficientUnits=N*m/(rad/s)  TorqueActuationMode=ComputedTorque  MotionActuationMode=InputMotion  SensePosition=on  SenseVelocity=off  SenseAcceleration=off  SenseTorqueForce=on  PositionTargetSpecify=off  PositionTargetPriority=High  PositionTargetValue=0  PositionTargetValueUnits=deg  VelocityTargetSpecify=off  VelocityTargetPriority=High  VelocityTargetValue=0  VelocityTargetValueUnits=deg/s
  link1 : Subsystem
  link2 : Subsystem
  link3 : Subsystem
  link4 : Subsystem
  link5 : Subsystem
  world_fixed : sm_lib/Joints/Weld Joint  SenseConstraintForce=off  SenseConstraintForceX=off  SenseConstraintForceY=off  SenseConstraintForceZ=off  SenseConstraintTorque=off  SenseConstraintTorqueX=off  SenseConstraintTorqueY=off  SenseConstraintTorqueZ=off  SenseTotalForce=off  SenseTotalForceX=off  SenseTotalForceY=off  SenseTotalForceZ=off  SenseTotalTorque=off  SenseTotalTorqueX=off  SenseTotalTorqueY=off  SenseTotalTorqueZ=off  CompositeWrenchDir=FollowerOnBase  CompositeWrenchFrame=BaseFrame
  W : PMIOPort  Port=1  Side=Left
  Bfa : PMIOPort  Port=2  Side=Right
  Bfb : PMIOPort  Port=3  Side=Right
  sensorData : Outport
  wires:
  Demux/3 -> Simulink-PS Converter3/1
  Demux/1 -> Simulink-PS Converter1/1
  Demux/2 -> Simulink-PS Converter2/1
  Demux/4 -> Simulink-PS Converter4/1
  Mux/1 -> sensorData/1
  Gain/1 -> Simulink-PS Converter5/1
  PS-Simulink Converter3/1 -> Mux/4  "Joint4Pos"
  Demux/5 -> Gain/1
  PS-Simulink Converter2/1 -> Mux/3  "Joint3Pos"
  PS-Simulink Converter1/1 -> Mux/2  "Joint2Pos"
  PS-Simulink Converter/1 -> Mux/1  "Joint1Pos"
  commands/1 -> Demux/1
  PS-Simulink Converter4/1 -> Terminator3/1  "J1 Torque"
  PS-Simulink Converter5/1 -> Terminator1/1  "J2 Torque"
  PS-Simulink Converter6/1 -> Terminator2/1  "J3 Torque"
  PS-Simulink Converter7/1 -> Terminator4/1  "J4 Torque"
  connections:
  grip_link/RConn1 -- Bfb/RConn1
  grip_link_sub/RConn1 -- Bfa/RConn1
  joint1/RConn2 -- PS-Simulink Converter/LConn1
  joint2/RConn2 -- PS-Simulink Converter1/LConn1
  joint1/LConn2 -- Simulink-PS Converter1/RConn1
  joint3/LConn2 -- Simulink-PS Converter3/RConn1
  joint4/LConn2 -- Simulink-PS Converter4/RConn1
  joint2/LConn2 -- Simulink-PS Converter2/RConn1
  joint4/RConn2 -- PS-Simulink Converter3/LConn1
  joint3/RConn2 -- PS-Simulink Converter2/LConn1
  grip_joint_sub/LConn2 -- Simulink-PS Converter5/RConn1 -- grip_joint/LConn2
  W/RConn1 -- world_fixed/LConn1
  Translational Hard Stop/RConn1 -- Translational Simscape Multibody1/RConn2
  MTRef/LConn1 -- Translational Hard Stop1/LConn1 -- Translational Simscape Multibody/LConn2
  Translational Hard Stop1/RConn1 -- Translational Simscape Multibody/RConn2
  MTRef1/LConn1 -- Translational Hard Stop/LConn1 -- Translational Simscape Multibody1/LConn2
  joint3/RConn1 -- link4/LConn1
  joint4/LConn1 -- link4/RConn1
  joint1/RConn1 -- link2/LConn1
  link1/LConn1 -- world_fixed/RConn1
  joint2/RConn1 -- link3/LConn1
  joint3/LConn1 -- link3/RConn1
  joint2/LConn1 -- link2/RConn1
  joint1/LConn1 -- link1/RConn1
  link5/RConn2 -- Translational Simscape Multibody1/LConn1 -- grip_joint/LConn1
  joint4/RConn1 -- link5/LConn1
  grip_link/LConn1 -- Translational Simscape Multibody1/RConn1 -- grip_joint/RConn1
  Translational Simscape Multibody/LConn1 -- link5/RConn1 -- grip_joint_sub/LConn1
  grip_link_sub/LConn1 -- Translational Simscape Multibody/RConn1 -- grip_joint_sub/RConn1
  joint1/RConn3 -- PS-Simulink Converter4/LConn1
  joint2/RConn3 -- PS-Simulink Converter5/LConn1
  joint3/RConn3 -- PS-Simulink Converter6/LConn1
  joint4/RConn3 -- PS-Simulink Converter7/LConn1

== system OpenManipulatorLib/Triggered Polynomial Fit ==
  Data : Inport
  Trigger : TriggerPort  VariantControl=Variant  PortDimensions=1
  Least Squares Polynomial Fit : dsppolyfun/Least Squares Polynomial Fit  X=linspace(0,estDelay,estDelay/Ts)  N=polyOrder
      settings: SourceProductName=DSP System Toolbox  SourceProductBaseCode=DS
  Coefficients : Outport
  wires:
  Least Squares Polynomial Fit/1 -> Coefficients/1
  Data/1 -> Least Squares Polynomial Fit/1

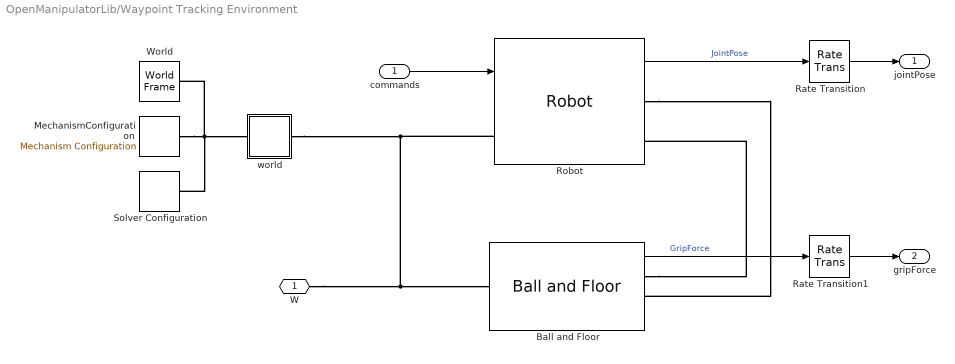
== system OpenManipulatorLib/Waypoint Tracking Environment ==
  commands : Inport
  Ball and Floor : OpenManipulatorLib/Ball and Floor  PxPositionTargetValue=initPosX  PyPositionTargetValue=initPosY  PxVelocityTargetValue=initVelX  PyVelocityTargetValue=initVelY  PzPositionTargetValue=initPosZ  PzVelocityTargetValue=initVelZ
  MechanismConfiguration : sm_lib/Utilities/Mechanism Configuration  UniformGravity=Constant  GravityVector=[0 0 -9.80665]  GravityUnits=m/s^2  LinearizationDelta=0.001
  Rate Transition : RateTransition
  Rate Transition1 : RateTransition
  Robot : OpenManipulatorLib/Robot  SystemSampleTime=-1
  Solver Configuration : nesl_utility/Solver Configuration  PhysicalDomain=network_engine_domain  SubClassName=solver  LeftPortType=input  RightPortType=generic  Accelerate=off  Tones=[]  Harmonics=[]  SimulateNoise=off  Profile=off  UseLocalSampling=off  EnableSwitchedLinearOptims=on  FrequencyDomain=off  UseCCode=off  RelTol=0.001  AbsTol=1e-06  MinStep=1e-09  ToWorkspace=off  RevertToSquareIcSolve=off  NumHomotopyIterations=100  PhasorMode=off  PhasorModeNumHarmonics=1  DoDC=off  ResidualTolerance=1e-09  UseLocalSolver=off  LocalSolverChoice=NE_BACKWARD_EULER_ADVANCER  LocalSolverSampleTime=0.001  DoFixedCost=off  MaxNonlinIter=3  MaxModeIter=2  LinearAlgebra=Sparse  DelaysMemoryBudget=1024  AutomaticFiltering=on  FilteringTimeConstant=0.001
  World : sm_lib/Frames and Transforms/World Frame
  world : Subsystem
  W : PMIOPort  Port=1  Side=Left
  jointPose : Outport
  gripForce : Outport  Port=2
  wires:
  commands/1 -> Robot/1
  Robot/1 -> Rate Transition/1  "JointPose"
  Ball and Floor/1 -> Rate Transition1/1  "GripForce"
  Rate Transition/1 -> jointPose/1
  Rate Transition1/1 -> gripForce/1
  connections:
  World/RConn1 -- MechanismConfiguration/RConn1 -- Solver Configuration/RConn1 -- world/LConn1
  W/RConn1 -- world/RConn1 -- Robot/LConn1 -- Ball and Floor/LConn1
  Ball and Floor/RConn1 -- Robot/RConn2
  Robot/RConn1 -- Ball and Floor/RConn2
